simulink model "D3_MPC_1_QuadrotorModel"  (R2023b)
settings: Solver=VariableStepAuto  StartTime=0.0  StopTime=60  FixedStep=0.0005  MaxStep=0.05  RelTol=1e-3
InitFcn:
  | nlobj = init_nmpc();
values from neighbouring files (symbols this model uses):
  A_flap = [c_a, c_b, 0 ... (first row only)    [LQR_calculate.m]    (also in LQR_feedback.m; LQR_linearized_test.m; MPC_test.m; MPC_test_1.m)
  A_ind = [c_d, 0, 0 ... (first row only)    [LQR_calculate.m]    (also in LQR_feedback.m; LQR_linearized_test.m; MPC_test.m; MPC_test_1.m)
  C_drag = 0    [LQR_calculate.m]    (also in LQR_feedback.m = C_drag_arr(i); LQR_linearized_test.m = C_drag_arr(i); MPC_test.m = C_drag_arr(i); MPC_test_1.m = C_drag_arr(i))
  demp = 0    [LQR_feedback.m]    (also in LQR_linearized_test.m; MPC_params.m; MPC_test_1.m; initQuadrotorData.m)
  forward_1 = 20    [LQR_feedback.m]    (also in LQR_linearized_test.m; MPC_test_1.m)
  forward_2 = 20    [LQR_feedback.m]    (also in LQR_linearized_test.m; MPC_test_1.m)
  g = 9.81    [LQR_calculate.m]    (also in LQR_feedback.m = 9.8; LQR_linearized_test.m = 9.8; LQR_testing_gpt.m; MPC_params.m = 9.8)
  Ix = m/3*a^2/12+2*0.045*l^2    (= 0.00211347222222)    [LQR_calculate.m]    (also in LQR_feedback.m; LQR_linearized_test.m; LQR_testing_gpt.m = 0.0081; MPC_params.m)
  Iy = m/3*a^2/12+4*0.045*l^2    (= 0.00413847222222)    [LQR_calculate.m]    (also in LQR_feedback.m = 0.00211347222222; LQR_linearized_test.m = 0.00211347222222; LQR_testing_gpt.m = 0.0081; MPC_params.m = 0.00211347222222)
  Iz = m/3*a^2/4+2*0.045*l^2    (= 0.00229041666667)    [LQR_calculate.m]    (also in LQR_feedback.m = 0.00431541666667; LQR_linearized_test.m = 0.00431541666667; LQR_testing_gpt.m = 0.0142; MPC_params.m = 0.00431541666667)
  J = 2.5*10^(-6)    (= 2.5e-06)    [LQR_calculate.m]    (also in LQR_feedback.m; LQR_linearized_test.m; MPC_params.m; MPC_test.m)
  Ke = ke    (= 0.0073)    [LQR_calculate.m]    (also in LQR_feedback.m = 0.00734; LQR_linearized_test.m = 0.00734; MPC_params.m = 0.00734; MPC_test.m)
  kf = ks*r^2*airDensity*Sblade/2    (= 1.57565625e-05)    [LQR_calculate.m]    (also in LQR_feedback.m; LQR_linearized_test.m; MPC_params.m; MPC_test.m)
  Km = kt    (= 0.0073)    [LQR_calculate.m]    (also in LQR_feedback.m = 0.00734; LQR_linearized_test.m = 0.00734; MPC_params.m = 0.00734; MPC_test.m)
  kv = 1300    [LQR_feedback.m]    (also in LQR_linearized_test.m; MPC_test_1.m; initQuadrotorData.m)
  L = La    (= 5e-05)    [LQR_calculate.m]    (also in LQR_feedback.m = 0.0001; LQR_linearized_test.m = 0.0001; MPC_params.m = 0.0001; MPC_test.m)
  l = 0.15    [LQR_calculate.m]    (also in LQR_feedback.m; LQR_linearized_test.m; MPC_params.m; MPC_test.m)
  m = size(B, 2)    [LQR_calculate.m]    (also in LQR_feedback.m = 0.65; LQR_linearized_test.m = 0.65; LQR_testing_gpt.m = 1; MPC_params.m = 0.65)
  maxU = 16    [LQR_calculate.m]    (also in LQR_feedback.m; LQR_linearized_test.m; MPC_params.m; MPC_test.m = 11)
  Mode = 3    [LQR_feedback.m]    (also in LQR_linearized_test.m; MPC_test_1.m = 1)
  N = params.N    [MPC_test_1.m]    (also in initQuadrotorData.m)
  phi0 = 0    [LQR_feedback.m]    (also in LQR_linearized_test.m; MPC_test_1.m)
  psi0 = pi/2    (= 1.57079632679)    [LQR_feedback.m]    (also in LQR_linearized_test.m; MPC_test_1.m = 0)
  Qc = diag([500, 500, 500, 1, 1, 1, 1, 1, 10, 1, 1, 1])    [MPC_test_1.m]
  R = eye(4)    [LQR_calculate.m]    (also in LQR_feedback.m = 0.058; LQR_linearized_test.m = 0.058; LQR_testing_gpt.m = diag([0.1, 10, 100, 10]); MPC_params.m = 0.058)
  Rc = diag([1, 1, 1, 1])    [LQR_feedback.m]    (also in LQR_linearized_test.m; MPC_test_1.m = diag([0.1, 0.1, 0.1, 0.1]))
  rho = 1.225    [LQR_calculate.m]    (also in LQR_feedback.m; LQR_linearized_test.m; MPC_params.m; MPC_test.m)
  S = l*c*4+a*b    (= 0.0169)    [LQR_calculate.m]    (also in LQR_feedback.m; LQR_linearized_test.m; MPC_params.m; MPC_test.m)
  theta0 = 0    [LQR_feedback.m]    (also in LQR_linearized_test.m; MPC_test_1.m)
  total_time = 60    [LQR_feedback.m]    (also in LQR_linearized_test.m; MPC_test_1.m)
  U_ref = repmat(u_nominal', params.N, 1)    [MPC_test_1.m]    (also in initQuadrotorData.m)
  up_down = 5    [LQR_feedback.m]    (also in LQR_linearized_test.m; MPC_test_1.m)
  x0 = 0    [LQR_feedback.m]    (also in LQR_linearized_test.m; MPC_test_1.m; init_nmpc.m = zeros(nx,1))
  y0 = 0    [LQR_feedback.m]    (also in LQR_linearized_test.m; MPC_test_1.m)
  z0 = 0    [LQR_feedback.m]    (also in LQR_linearized_test.m; MPC_test_1.m)
libraries: vrlib x2, mpclib x1, sharedtransform x1
(part 2 of 2)

== matlab function D3_MPC_1_QuadrotorModel/MATLAB Function7 ==
  data: eul input; axisAngle output
function axisAngle = eul2AxisAngle(eul)
% eul: [phi; theta; psi] – углы Эйлера в радианах (roll, pitch, yaw)
% axisAngle: [ax; ay; az; angle] – axis‑angle, угол в рад

    % Конвертируем сначала в кватернион [w x y z]
    % MATLAB ожидает порядок [yaw pitch roll] и стандарт 'ZYX'
    q = eul2quat([eul(3), eul(2), eul(1)], 'ZYX');  
    
    % Вычисляем угол поворота
    angle = 2 * acos( q(1) );
    
    % sin(theta/2) для нормировки оси
    s = sqrt(1 - q(1)^2);
    
    if s < 1e-6
        % Угол почти нулевой — ось можно задать произвольно
        axis = [1; 0; 0];
    else
        % Нормируем вектор-проекция кватерниона
        axis = q(2:4)' / s;
    end
    
    axisAngle = [axis; angle];
end

== matlab function D3_MPC_1_QuadrotorModel/MATLAB Function8 ==
  data: t input; rot output
function rot = rotor_angle(t)
%#codegen
    omega = 20; % рад/с
    angle = mod(omega * t, 2*pi);
    rot = [0 0 1 angle];  % вращение вокруг оси Z
end
